simulink model "Buck_w_PI_Controller"  (R2023b)
settings: Solver=ode45  StartTime=0.0  StopTime=2.5e-5*400  MaxStep=1e-7  RelTol=1e-5
libraries: spsSeriesRLCBranchLib x3, simulink x2, spsCurrentMeasurementLib x1, spsControlledVoltageSourceLib x1, spsDiodeLib x1, spsMosfetLib x1, spsVoltageMeasurementLib x1, sps_lib x1
settings Model: Creator=jiaxinteng  LastModifiedBy=Dajr
settings SolverCC: AlgebraicLoopSolver=TrustRegion
settings DataIOCC: ReturnWorkspaceOutputs=off
settings OptimizationCC: LifeSpan=inf
settings DebuggingCC: UnconnectedInputMsg=warning  UnconnectedOutputMsg=warning  UnconnectedLineMsg=warning  SFExecutionAtInitializationDiag=none  ArithmeticOperatorsInVariantConditions=warning
settings HardwareCC: ProdBitPerSizeT=32  ProdBitPerPtrDiffT=32  ProdWordSize=32  ProdHWDeviceType=Specified
settings ModelReferenceCC: EnableRefExpFcnMdlSchedulingChecks=on
settings SFSimCC: SimUseLocalCustomCode=off  CustomCodeUndefinedFunction=UseInterfaceOnly
settings RTWCC: RTWUseLocalCustomCode=off
settings CodeAppCC: StateflowObjectComments=on
settings SimscapeCC: SimscapeNormalizeSystem=off
settings ConfigurationSet: Description=SimMechanics 2G

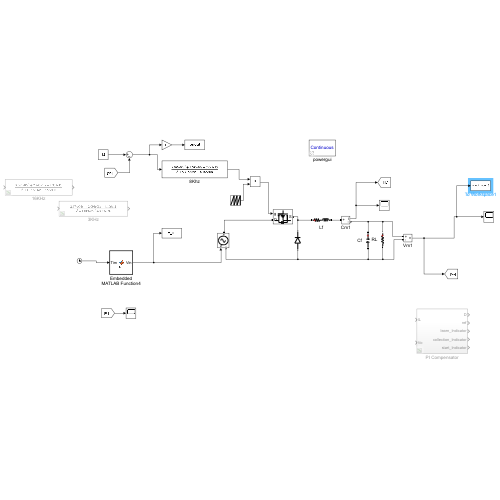
[thumbnail: Simulink's stored preview of the top-level diagram]
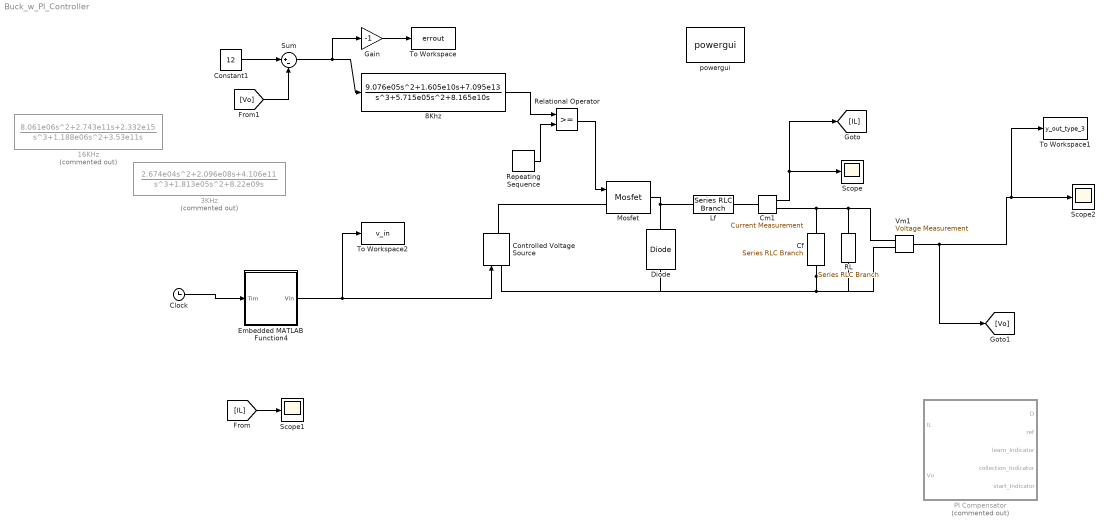
== system Buck_w_PI_Controller ==
  16KHz : TransferFcn  Commented=on  Numerator=[8.061e06 2.743e11 2.332e15]  Denominator=[1 1.188e06 3.53e11 0]
  3KHz : TransferFcn  Commented=on  Numerator=[2.674e04 2.096e08 4.106e11]  Denominator=[1 1.813e05 8.22e09 0]
  8Khz : TransferFcn  Numerator=[9.076e05 1.605e10 7.095e13]  Denominator=[1 5.715e05 8.165e10 0]
  Cf : spsSeriesRLCBranchLib/Series RLC Branch  LConnTagsString=__new0  RConnTagsString=__new0  BranchType=C  Resistance=20e-3  Inductance=220e-6  SetiL0=off  InitialCurrent=0  Capacitance=50e-6  Setx0=off  InitialVoltage=7  Measurements=None
  Clock : Clock
  Cm1 : spsCurrentMeasurementLib/Current Measurement  PhasorSimulation=off  OutputType=Complex  PSBequivalent=0
  Constant1 : Constant  Value=12
  Controlled Voltage Source : spsControlledVoltageSourceLib/Controlled Voltage Source  Initialize=on  Source_Type=AC  Amplitude=0  Phase=0  Frequency=0  Measurements=None
  Diode : spsDiodeLib/Diode  Ron=0.001  Lon=0  Vf=0.8  IC=0  UseSnubber=off  Rs=500  Cs=250e-9  Measurements=off
  Embedded MATLAB Function4 : MATLAB Function  TreatAsAtomicUnit=on  SystemSampleTime=2.5e-5
  Gain : Gain  Gain=-1
  Lf : spsSeriesRLCBranchLib/Series RLC Branch  LConnTagsString=__new0  RConnTagsString=__new0  BranchType=RL  Resistance=0.1  Inductance=220e-6  SetiL0=off  InitialCurrent=0  Capacitance=1e-6  Setx0=off  InitialVoltage=0  Measurements=None
  Mosfet : spsMosfetLib/Mosfet  Ron=0.1  Lon=0  Rd=0.01  Vfd=0  IC=0  Rs=1e5  Cs=inf  Measurements=off
  PI Compensator : Subsystem  Commented=on
  RL : spsSeriesRLCBranchLib/Series RLC Branch  LConnTagsString=__new0  RConnTagsString=__new0  BranchType=R  Resistance=10  Inductance=220e-6  SetiL0=off  InitialCurrent=0  Capacitance=50e-6  Setx0=off  InitialVoltage=0  Measurements=None
  Relational Operator : RelationalOperator  OutDataTypeStr=boolean  RndMeth=Simplest  InputSameDT=off
  Repeating Sequence : simulink/Sources/Repeating Sequence  rep_seq_t=[0 1/160000]  rep_seq_y=[0 1]
  Scope : Scope
  Scope1 : Scope
  Scope2 : Scope
  Sum : Sum  Inputs=|+-
  To Workspace : ToWorkspace  VariableName=errout  SaveFormat=Timeseries  SampleTime=-1
  To Workspace1 : ToWorkspace  VariableName=y_out_type_3  SaveFormat=Timeseries  SampleTime=-1
  To Workspace2 : ToWorkspace  VariableName=v_in  SaveFormat=Timeseries  SampleTime=-1
  Vm1 : spsVoltageMeasurementLib/Voltage Measurement  PhasorSimulation=off  OutputType=Complex  PSBequivalent=0
  powergui : sps_lib/powergui  Priority=1  SimulationMode=Continuous  SampleTime=1e-7  frequency=60  Iterations=50  frequencyindice=0  Pbase=100e6  ErrMax=1e-4  UnitsV=kV  UnitsW=MW  buscounter=0  FunctionMessages=off  echomessages=off  EnableUseOfTLC=off  CurrentSourceSwitches=off  DisableSnubberDevices=on  DisableRonSwitches=on  DisableVfSwitches=on  DisplayEquations=off  AutomaticDiscreteSolvers=off  SolverType=Tustin/Backward Euler (TBE)  Interpol=off  ExternalGateDelay=off  methode=off  Ts=10  x0status=blocks  SPID=off  SwTol=0  HookPort=off  NonlinearTolerance=1e-4  nMaxIteration=100  ContinueOnMaxIteration=off  RestoreLinks=warning  ResistiveCurrentMeasurement=off  Frange=[0:2:500]  Ylog=off  Xlog=on  ShowGrid=off  save=off  variable=ZData  structure=x1  ZoomFFT=off  StartTime=0.0  cycles=1  DisplayStyle=1  fundamental=80e3  FreqAxis=off  MaxFrequency=100e3  frequencyindicesteady=1  RmsSteady=1  display=off
  wires:
  Cm1/1 -> [IL], Scope/1
  Vm1/1 -> [Vo], To Workspace1/1, Scope2/1
  Clock/1 -> Embedded MATLAB Function4/1(Tim)
  Embedded MATLAB Function4/1(Vin) -> To Workspace2/1, Controlled Voltage Source/1
  [IL] -> Scope1/1
  Constant1/1 -> Sum/1
  [Vo] -> Sum/2
  Sum/1 -> 8Khz/1, Gain/1
  8Khz/1 -> Relational Operator/1
  Repeating Sequence/1 -> Relational Operator/2
  Relational Operator/1 -> Mosfet/1
  Gain/1 -> To Workspace/1
  connections:
  Diode/RConn1 -- Lf/LConn1 -- Mosfet/RConn1
  Vm1/LConn1 -- RL/LConn1 -- Cm1/RConn1 -- Cf/LConn1
  Cf/RConn1 -- Vm1/LConn2 -- RL/RConn1 -- Controlled Voltage Source/LConn1 -- Diode/LConn1
  Cm1/LConn1 -- Lf/RConn1
  Mosfet/LConn1 -- Controlled Voltage Source/RConn1

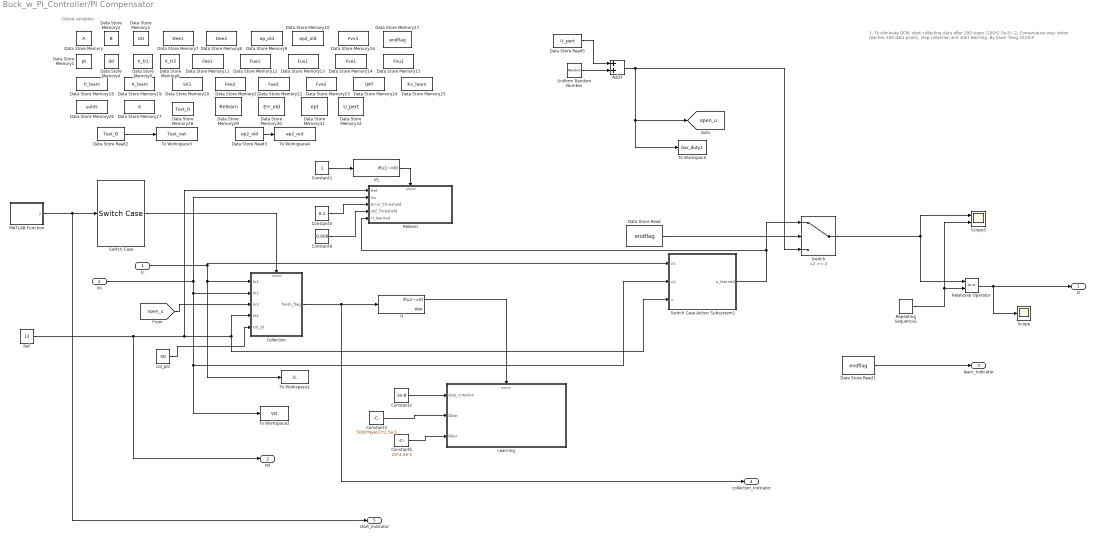
== system Buck_w_PI_Controller/PI Compensator ==
  note: Global variables:
  note: 1. To eliminate DCM, start collecting data after 200 steps (200*2.5e-5),
      | 2. Conservative way: when reaches 100 data points, stop collection and start learning.
      |
      | By Jiaxin Teng
      | 2019.8
  IL : Inport
  Vo : Inport  Port=2
  Add3 : Sum
  Collection : Subsystem  TreatAsAtomicUnit=on
  Constant1 : Constant
  Constant2 : Constant  Value=1e-8
  Constant3 : Constant  Value=5000*eye(2)*2.5e-5
  Constant4 : Constant  Value=20*2.5e-5
  Constant5 : Constant  Value=0.1
  Constant6 : Constant  Value=0.008
  Data Store Memory : DataStoreMemory  ReadBeforeWriteMsg=warning  WriteAfterWriteMsg=warning  WriteAfterReadMsg=warning  InitialValue=zeros(50,1)  ShowAdditionalParam=off  OutDataTypeStr=double
  Data Store Memory1 : DataStoreMemory  DataStoreName=pt  ReadBeforeWriteMsg=warning  WriteAfterWriteMsg=warning  WriteAfterReadMsg=warning  InitialValue=1  ShowAdditionalParam=off  OutDataTypeStr=double
  Data Store Memory10 : DataStoreMemory  DataStoreName=ep2_old  ReadBeforeWriteMsg=warning  WriteAfterWriteMsg=warning  WriteAfterReadMsg=warning  InitialValue=zeros(1,2)  VectorParams1D=off  ShowAdditionalParam=off  OutDataTypeStr=double
  Data Store Memory11 : DataStoreMemory  DataStoreName=Fee1  ReadBeforeWriteMsg=warning  WriteAfterWriteMsg=warning  WriteAfterReadMsg=warning  InitialValue=zeros(50,4)  ShowAdditionalParam=off  OutDataTypeStr=double
  Data Store Memory12 : DataStoreMemory  DataStoreName=Fue1  ReadBeforeWriteMsg=warning  WriteAfterWriteMsg=warning  WriteAfterReadMsg=warning  InitialValue=zeros(50,2)  ShowAdditionalParam=off  OutDataTypeStr=double
  Data Store Memory13 : DataStoreMemory  DataStoreName=Fuu1  ReadBeforeWriteMsg=warning  WriteAfterWriteMsg=warning  WriteAfterReadMsg=warning  InitialValue=zeros(50,1)  ShowAdditionalParam=off  OutDataTypeStr=double
  Data Store Memory14 : DataStoreMemory  DataStoreName=Fve1  ReadBeforeWriteMsg=warning  WriteAfterWriteMsg=warning  WriteAfterReadMsg=warning  InitialValue=zeros(50,2)  ShowAdditionalParam=off  OutDataTypeStr=double
  Data Store Memory15 : DataStoreMemory  DataStoreName=Fvu1  ReadBeforeWriteMsg=warning  WriteAfterWriteMsg=warning  WriteAfterReadMsg=warning  InitialValue=zeros(50,1)  ShowAdditionalParam=off  OutDataTypeStr=double
  Data Store Memory16 : DataStoreMemory  DataStoreName=Fvv1  ReadBeforeWriteMsg=warning  WriteAfterWriteMsg=warning  WriteAfterReadMsg=warning  InitialValue=zeros(50,1)  ShowAdditionalParam=off  OutDataTypeStr=double
  Data Store Memory17 : DataStoreMemory  DataStoreName=endflag  ReadBeforeWriteMsg=warning  WriteAfterWriteMsg=warning  WriteAfterReadMsg=warning  ShowAdditionalParam=off  OutDataTypeStr=double
  Data Store Memory18 : DataStoreMemory  DataStoreName=P_learn  ReadBeforeWriteMsg=warning  WriteAfterWriteMsg=warning  WriteAfterReadMsg=warning  InitialValue=zeros(2,2)  ShowAdditionalParam=off  OutDataTypeStr=double
  Data Store Memory19 : DataStoreMemory  DataStoreName=K_learn  ReadBeforeWriteMsg=warning  WriteAfterWriteMsg=warning  WriteAfterReadMsg=warning  InitialValue=zeros(1,2)  VectorParams1D=off  ShowAdditionalParam=off  OutDataTypeStr=double
  Data Store Memory2 : DataStoreMemory  DataStoreName=B  ReadBeforeWriteMsg=warning  WriteAfterWriteMsg=warning  WriteAfterReadMsg=warning  InitialValue=zeros(50,1)  ShowAdditionalParam=off  OutDataTypeStr=double
  Data Store Memory20 : DataStoreMemory  DataStoreName=SX1  ReadBeforeWriteMsg=warning  WriteAfterWriteMsg=warning  WriteAfterReadMsg=warning  InitialValue=zeros(2,1)  ShowAdditionalParam=off  OutDataTypeStr=double
  Data Store Memory21 : DataStoreMemory  DataStoreName=Fee2  ReadBeforeWriteMsg=warning  WriteAfterWriteMsg=warning  WriteAfterReadMsg=warning  InitialValue=zeros(50,4)  ShowAdditionalParam=off  OutDataTypeStr=double
  Data Store Memory22 : DataStoreMemory  DataStoreName=Fue2  ReadBeforeWriteMsg=warning  WriteAfterWriteMsg=warning  WriteAfterReadMsg=warning  InitialValue=zeros(50,2)  ShowAdditionalParam=off  OutDataTypeStr=double
  Data Store Memory23 : DataStoreMemory  DataStoreName=Fve2  ReadBeforeWriteMsg=warning  WriteAfterWriteMsg=warning  WriteAfterReadMsg=warning  InitialValue=zeros(50,2)  ShowAdditionalParam=off  OutDataTypeStr=double
  Data Store Memory24 : DataStoreMemory  DataStoreName=QKf  ReadBeforeWriteMsg=warning  WriteAfterWriteMsg=warning  WriteAfterReadMsg=warning  InitialValue=zeros(2,2)  ShowAdditionalParam=off  OutDataTypeStr=double
  Data Store Memory25 : DataStoreMemory  DataStoreName=Kv_learn  ReadBeforeWriteMsg=warning  WriteAfterWriteMsg=warning  WriteAfterReadMsg=warning  ShowAdditionalParam=off  OutDataTypeStr=double
  Data Store Memory26 : DataStoreMemory  DataStoreName=sol45  ReadBeforeWriteMsg=warning  WriteAfterWriteMsg=warning  WriteAfterReadMsg=warning  InitialValue=zeros(2,1)  ShowAdditionalParam=off  OutDataTypeStr=double
  Data Store Memory27 : DataStoreMemory  DataStoreName=K  ReadBeforeWriteMsg=warning  WriteAfterWriteMsg=warning  WriteAfterReadMsg=warning  InitialValue=[0.2,0.2]  VectorParams1D=off  ShowAdditionalParam=off  OutDataTypeStr=double
  Data Store Memory28 : DataStoreMemory  DataStoreName=Test_D  ReadBeforeWriteMsg=warning  WriteAfterWriteMsg=warning  WriteAfterReadMsg=warning  InitialValue=zeros(50,4)  ShowAdditionalParam=off  OutDataTypeStr=double
  Data Store Memory29 : DataStoreMemory  DataStoreName=Relearn  ReadBeforeWriteMsg=warning  WriteAfterWriteMsg=warning  WriteAfterReadMsg=warning  ShowAdditionalParam=off  OutDataTypeStr=double
  Data Store Memory3 : DataStoreMemory  DataStoreName=UU  ReadBeforeWriteMsg=warning  WriteAfterWriteMsg=warning  WriteAfterReadMsg=warning  InitialValue=zeros(50,1)  ShowAdditionalParam=off  OutDataTypeStr=double
  Data Store Memory30 : DataStoreMemory  DataStoreName=Err_old  ReadBeforeWriteMsg=warning  WriteAfterWriteMsg=warning  WriteAfterReadMsg=warning  InitialValue=zeros(1000,1)  ShowAdditionalParam=off  OutDataTypeStr=double
  Data Store Memory31 : DataStoreMemory  DataStoreName=ept  ReadBeforeWriteMsg=warning  WriteAfterWriteMsg=warning  WriteAfterReadMsg=warning  InitialValue=1  ShowAdditionalParam=off  OutDataTypeStr=double
  Data Store Memory32 : DataStoreMemory  DataStoreName=U_pert  ReadBeforeWriteMsg=warning  WriteAfterWriteMsg=warning  WriteAfterReadMsg=warning  InitialValue=0.32  ShowAdditionalParam=off  OutDataTypeStr=double
  Data Store Memory4 : DataStoreMemory  DataStoreName=dd  ReadBeforeWriteMsg=warning  WriteAfterWriteMsg=warning  WriteAfterReadMsg=warning  InitialValue=1  ShowAdditionalParam=off  OutDataTypeStr=uint8
  Data Store Memory5 : DataStoreMemory  DataStoreName=X_tr1  ReadBeforeWriteMsg=warning  WriteAfterWriteMsg=warning  WriteAfterReadMsg=warning  InitialValue=[0;1]  ShowAdditionalParam=off  OutDataTypeStr=double
  Data Store Memory6 : DataStoreMemory  DataStoreName=X_tr2  ReadBeforeWriteMsg=warning  WriteAfterWriteMsg=warning  WriteAfterReadMsg=warning  InitialValue=[1;0]  ShowAdditionalParam=off  OutDataTypeStr=double
  Data Store Memory7 : DataStoreMemory  DataStoreName=Dee1  ReadBeforeWriteMsg=warning  WriteAfterWriteMsg=warning  WriteAfterReadMsg=warning  InitialValue=zeros(50,3)  ShowAdditionalParam=off  OutDataTypeStr=double
  Data Store Memory8 : DataStoreMemory  DataStoreName=Dee2  ReadBeforeWriteMsg=warning  WriteAfterWriteMsg=warning  WriteAfterReadMsg=warning  InitialValue=zeros(50,3)  ShowAdditionalParam=off  OutDataTypeStr=double
  Data Store Memory9 : DataStoreMemory  DataStoreName=ep_old  ReadBeforeWriteMsg=warning  WriteAfterWriteMsg=warning  WriteAfterReadMsg=warning  InitialValue=zeros(1,2)  VectorParams1D=off  ShowAdditionalParam=off  OutDataTypeStr=double
  Data Store Read : DataStoreRead  DataStoreName=endflag  IndexOptions=Index vector (dialog)  Indices=1  OutputSizes=1
  Data Store Read1 : DataStoreRead  DataStoreName=endflag  IndexOptions=Index vector (dialog)  Indices=1  OutputSizes=1
  Data Store Read2 : DataStoreRead  DataStoreName=Test_D  IndexOptions=Index vector (dialog)  Indices=1  OutputSizes=1
  Data Store Read3 : DataStoreRead  DataStoreName=ep2_old  IndexOptions=Index vector (dialog)  Indices=1  OutputSizes=1
  Data Store Read5 : DataStoreRead  DataStoreName=U_pert  IndexOptions=Index vector (dialog)  Indices=1  OutputSizes=1
  If : If  IfExpression=u1~=0
  If1 : If  IfExpression=u1~=0  ShowElse=off
  Learning : Subsystem  TreatAsAtomicUnit=on
  MATLAB Function : MATLAB Function  TreatAsAtomicUnit=on  SystemSampleTime=2.5e-5
  Ref : Constant  Value=12
  Relational Operator : RelationalOperator  OutDataTypeStr=boolean  InputSameDT=off
  Relearn : Subsystem
  Repeating Sequence1 : simulink/Sources/Repeating Sequence  rep_seq_t=[0 1/(160e3) 1/(80e3)]  rep_seq_y=[0 1 0]
  Scope : Scope
  Scope3 : Scope  NumInputPorts=2
  Switch : Switch  Threshold=2  SaturateOnIntegerOverflow=off  InputSameDT=off
  Switch Case : SwitchCase  CaseConditions={1,2}
  Switch Case Action Subsystem1 : Subsystem  TreatAsAtomicUnit=on
  To Workspace : ToWorkspace  VariableName=bar_duty1  SaveFormat=Structure With Time  SampleTime=2.5e-5
  To Workspace1 : ToWorkspace  VariableName=IL  SaveFormat=Structure With Time  SampleTime=2.5e-5
  To Workspace2 : ToWorkspace  VariableName=VO  SaveFormat=Structure With Time  SampleTime=2.5e-5
  To Workspace3 : ToWorkspace  VariableName=Test_out  SaveFormat=Timeseries  SampleTime=-1
  To Workspace4 : ToWorkspace  VariableName=ep2_out  SaveFormat=Timeseries  SampleTime=-1
  Uniform Random Number : UniformRandomNumber  Minimum=-5e-3  Maximum=5e-3  SampleTime=2.5e-5
  col_pts : Constant  Value=50
  D : Outport
  ref : Outport  Port=2
  learn_Indicator : Outport  Port=3
  collection_Indicator : Outport  Port=4
  start_Indicator : Outport  Port=5
  tag scope: open_u=global
  wires:
  Relational Operator/1 -> D/1, Scope/1
  Repeating Sequence1/1 -> Scope3/2, Relational Operator/2
  IL/1 -> To Workspace1/1, Collection/1(In1), Switch Case Action Subsystem1/1(x1)
  Vo/1 -> To Workspace2/1, Switch Case Action Subsystem1/2(x2), Collection/2(In2), Relearn/2(Vo)
  Collection/1(finish_flag) -> collection_Indicator/1, If/1
  If/1 -> Learning/Action
  [open_u] -> Collection/3(In3)
  Switch Case/2 -> Collection/Action
  MATLAB Function/1(y) -> start_Indicator/1, Switch Case/1
  Constant2/1 -> Learning/1(stop_criterion)
  Constant3/1 -> Learning/2(Qbar)
  Constant4/1 -> Learning/3(Rbar)
  Data Store Read/1 -> Switch/2
  Switch Case Action Subsystem1/1(u_learned) -> Relearn/5(U_learned), Switch/1
  Add3/1 -> [open_u], To Workspace/1, Switch/3
  Switch/1 -> Scope3/1, Relational Operator/1
  Data Store Read5/1 -> Add3/1
  Uniform Random Number/1 -> Add3/2
  Data Store Read1/1 -> learn_Indicator/1
  Data Store Read3/1 -> To Workspace4/1
  Data Store Read2/1 -> To Workspace3/1
  Constant5/1 -> Relearn/3(Error_Threshold)
  Constant6/1 -> Relearn/4(std_Threshold)
  Ref/1 -> ref/1, Relearn/1(Ref), Collection/4(In4), Switch Case Action Subsystem1/3(v)
  If1/1 -> Relearn/Action
  Constant1/1 -> If1/1
  col_pts/1 -> Collection/5(col_pt)

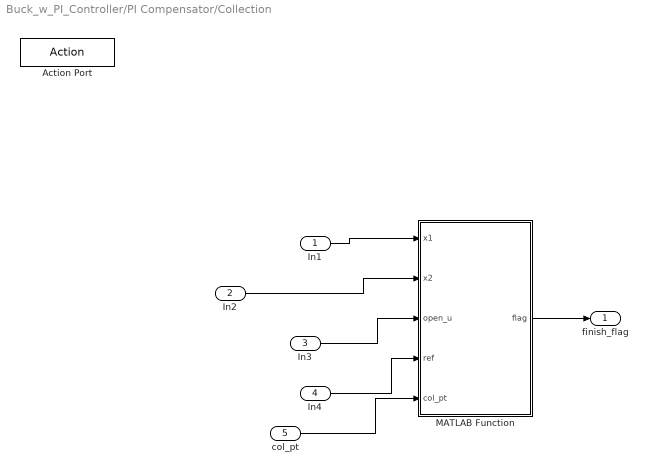
== system Buck_w_PI_Controller/PI Compensator/Collection ==
  In1 : Inport
  In2 : Inport  Port=2
  In3 : Inport  Port=3
  In4 : Inport  Port=4
  col_pt : Inport  Port=5
  Action Port : ActionPort  ActionPortLabel=case [ 2 ]:
  MATLAB Function : MATLAB Function  TreatAsAtomicUnit=on  SystemSampleTime=2.5e-5
  finish_flag : Outport
  wires:
  In1/1 -> MATLAB Function/1(x1)
  In2/1 -> MATLAB Function/2(x2)
  In3/1 -> MATLAB Function/3(open_u)
  MATLAB Function/1(flag) -> finish_flag/1
  In4/1 -> MATLAB Function/4(ref)
  col_pt/1 -> MATLAB Function/5(col_pt)

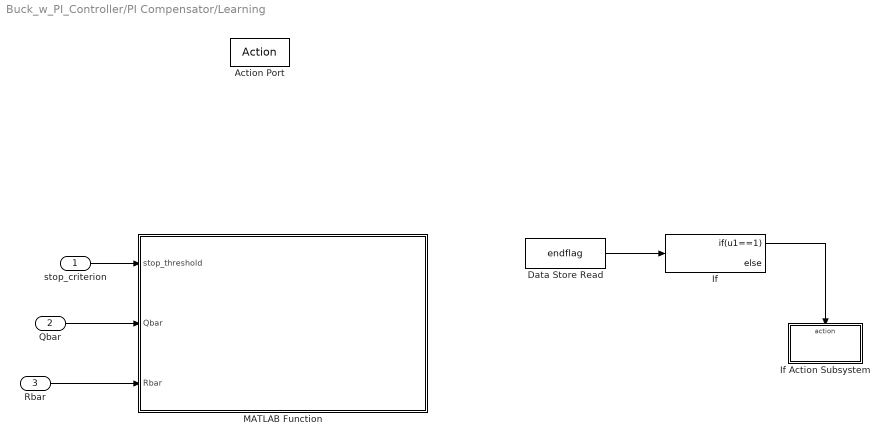
== system Buck_w_PI_Controller/PI Compensator/Learning ==
  stop_criterion : Inport
  Qbar : Inport  Port=2
  Rbar : Inport  Port=3
  Action Port : ActionPort  ActionPortLabel=if(u1~=0)
  Data Store Read : DataStoreRead  DataStoreName=endflag  IndexOptions=Index vector (dialog)  Indices=1  OutputSizes=1
  If : If  IfExpression=u1==1
  If Action Subsystem : Subsystem  TreatAsAtomicUnit=on
  MATLAB Function : MATLAB Function  TreatAsAtomicUnit=on
  wires:
  stop_criterion/1 -> MATLAB Function/1(stop_threshold)
  Data Store Read/1 -> If/1
  If/1 -> If Action Subsystem/Action
  Qbar/1 -> MATLAB Function/2(Qbar)
  Rbar/1 -> MATLAB Function/3(Rbar)

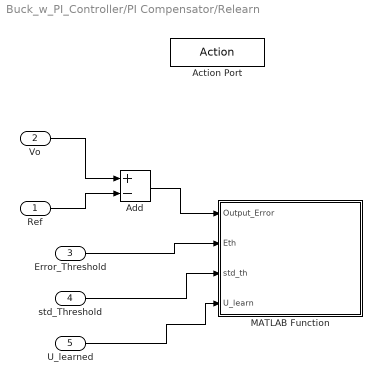
== system Buck_w_PI_Controller/PI Compensator/Relearn ==
  Ref : Inport
  Vo : Inport  Port=2
  Error_Threshold : Inport  Port=3
  std_Threshold : Inport  Port=4
  U_learned : Inport  Port=5
  Action Port : ActionPort  ActionPortLabel=if(u1~=0)
  Add : Sum  Inputs=+-
  MATLAB Function : MATLAB Function  TreatAsAtomicUnit=on
  wires:
  Error_Threshold/1 -> MATLAB Function/2(Eth)
  std_Threshold/1 -> MATLAB Function/3(std_th)
  Ref/1 -> Add/2
  Vo/1 -> Add/1
  Add/1 -> MATLAB Function/1(Output_Error)
  U_learned/1 -> MATLAB Function/4(U_learn)

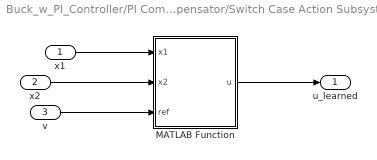
== system Buck_w_PI_Controller/PI Compensator/Switch Case Action Subsystem1 ==
  x1 : Inport
  x2 : Inport  Port=2
  v : Inport  Port=3
  MATLAB Function : MATLAB Function  TreatAsAtomicUnit=on  SystemSampleTime=2.5e-5
  u_learned : Outport
  wires:
  x1/1 -> MATLAB Function/1(x1)
  x2/1 -> MATLAB Function/2(x2)
  v/1 -> MATLAB Function/3(ref)
  MATLAB Function/1(u) -> u_learned/1

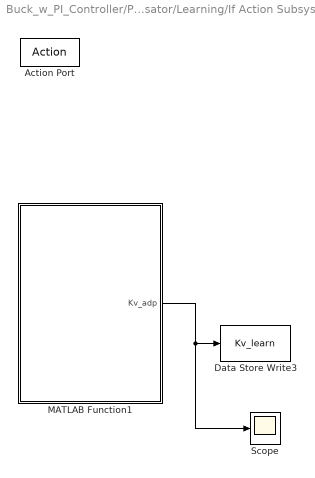
== system Buck_w_PI_Controller/PI Compensator/Learning/If Action Subsystem ==
  Action Port : ActionPort  ActionPortLabel=if(u1==1)
  Data Store Write3 : DataStoreWrite  DataStoreName=Kv_learn  IndexOptions=Index vector (dialog)  Indices=1  OutputSizes=1
  MATLAB Function1 : MATLAB Function  TreatAsAtomicUnit=on
  Scope : Scope
  wires:
  MATLAB Function1/1(Kv_adp) -> Scope/1, Data Store Write3/1

== matlab function Buck_w_PI_Controller/PI Compensator/Learning/If Action Subsystem/MATLAB Function1 ==
  data: Dee1 data_store_memory; Dee2 data_store_memory; Fee2 data_store_memory; Fue2 data_store_memory; Fve2 data_store_memory; Fvu1 data_store_memory; Fuu1 data_store_memory; Fvv1 data_store_memory; Kv_adp output; endflag data_store_memory; QKf data_store_memory; X_tr1 data_store_memory; X_tr2 data_store_memory; K_learn data_store_memory; SX1 data_store_memory; sol45 data_store_memory
function Kv_adp  = fcn
global Dee2 Fee2 Fue2 Fve2 Fvu1 Fuu1 Fvv1 K_learn SX1 endflag QKf X_tr1 X_tr2 sol45


    phi12=Dee2(2:end,:);
    Y2=Fee2(1:end-1,:)*QKf(:); 
    phi22=-2*((Fee2(1:end-1,:)*kron(K_learn',eye(2)))+Fue2(1:end-1,:));
    phi32=-Fuu1(1:end-1,:)+Fee2(1:end-1,:)*kron(K_learn',K_learn');
    phi42=-Fvv1(1:end-1,:);
    phi52=2*Fve2(1:end-1,:);
    phi62=2*Fvu1(1:end-1);
    X2=[phi12 phi22 phi32 phi42 phi52 phi62];
    sol2=(X2'*X2)\X2'*Y2;
    SX2=sol2(8:9);
    
    AA=[SX2(:) zeros(2,2) -sol45;
    X_tr2 -eye(2,2) zeros(2,1)];
    BB=[-SX1(:); -X_tr1];
    RegSol=AA\BB;
    Xreal=RegSol(2:3);
    Ureal=RegSol(4);
    Kv_adp=Ureal+K_learn*Xreal;
    endflag=2;


end

== matlab function Buck_w_PI_Controller/PI Compensator/Switch Case Action Subsystem1/MATLAB Function ==
  data: x1 input; u output; x2 input; ref input; K_learn data_store_memory; Kv_learn data_store_memory
function u = fcn(x1,x2,ref)
global K_learn Kv_learn

u=-K_learn*[x1;x2]+Kv_learn*ref;

if(u>1)
    u=1;
elseif(u<0)
    u=0;
end

end

== matlab function Buck_w_PI_Controller/PI Compensator/Relearn/MATLAB Function ==
  data: Output_Error input; Eth input; std_th input; endflag data_store_memory; pt data_store_memory; ept data_store_memory; Relearn data_store_memory; Err_old data_store_memory; U_learn input; U_pert data_store_memory
function fcn(Output_Error, Eth, std_th, U_learn)
global endflag pt Relearn Err_old ept U_pert

Err_old(ept) = Output_Error;
ept = ept+1;
if ept>(length(Err_old))
    ept=ept-(length(Err_old));
end
err_mean = mean(Err_old);
err_std = std(Err_old);

if ( (abs(err_mean) > Eth) && (err_std < std_th) ) && ( (endflag == 2)&& (Relearn == 0) )
    U_pert = U_learn;
    pt=1;
    endflag=0;

end

end

== matlab function Buck_w_PI_Controller/Embedded MATLAB Function4 ==
  data: Vin output; Tim input
function Vin = fcn(Tim)  

Vin=40;

% if (Tim>0.009)&&(Tim<0.01275)
%     Vin=48;
% elseif (Tim>=0.01275)&&(Tim<0.0163)
%     Vin=60;
% elseif (Tim>=0.0163)
%     Vin=36;
% end

end

== matlab function Buck_w_PI_Controller/PI Compensator/Learning/MATLAB Function ==
  data: Dee1 data_store_memory; Dee2 data_store_memory; Fee1 data_store_memory; Fue1 data_store_memory; Fve1 data_store_memory; Fvu1 data_store_memory; Fuu1 data_store_memory; Fvv1 data_store_memory; endflag data_store_memory; stop_threshold input; QKf data_store_memory; sol45 data_store_memory; P_learn data_store_memory; K_learn data_store_memory; SX1 data_store_memory; Qbar input; Rbar input; K data_store_memory
function fcn(stop_threshold,Qbar,Rbar)
global Dee1 Fee1 Fue1 Fve1 Fvu1 Fuu1 Fvv1 endflag QKf sol45 P_learn K_learn SX1 K
    
phi1=Dee1(2:end,:); Pp=zeros(2); 


%for m=1:50
while endflag==0
QK=-Qbar-K'*Rbar*K;

phi2=-2*((Fee1(1:end-1,:)*kron(K',eye(2)))+Fue1(1:end-1,:));
phi3=-Fuu1(1:end-1)+Fee1(1:end-1,:)*kron(K',K');
phi4=-Fvv1(1:end-1);
phi5=2*Fve1(1:end-1,:);
phi6=2*Fvu1(1:end-1);

X=[phi1 phi2 phi3 phi4 phi5 phi6];

% RANK=rank(X);
    
Y=Fee1(1:end-1,:)*QK(:);

sol=(X'*X)\X'*Y;

P=[sol(1) sol(2)/2; sol(2)/2 sol(3)];
K=(Rbar+sol(6))\sol(4:5)';

if(norm(P-Pp)<stop_threshold)
    P_learn=P; K_learn=K; SX1=sol(8:9); QKf=-Qbar-K'*Rbar*K; sol45=sol(4:5);
    endflag=1;
else 
    endflag=0;
end

Pp=P;

end

end

== matlab function Buck_w_PI_Controller/PI Compensator/Collection/MATLAB Function ==
  data: x1 input; pt data_store_memory; A data_store_memory; flag output; x2 input; B data_store_memory; open_u input; UU data_store_memory; X_tr1 data_store_memory; X_tr2 data_store_memory; Dee1 data_store_memory; Dee2 data_store_memory; ref input; ep_old data_store_memory; ep2_old data_store_memory; Fee1 data_store_memory; Fue1 data_store_memory; Fve1 data_store_memory; Fvu1 data_store_memory; Fuu1 data_store_memory; Fvv1 data_store_memory; Fee2 data_store_memory; Fve2 data_store_memory; Fue2 data_store_memory; Test_D data_store_memory; Relearn data_store_memory; col_pt input
function flag=fcn(x1,x2,open_u,ref, col_pt)
global A B UU pt X_tr1 X_tr2 Dee1 Dee2 Fee1 Fee2 Fue1 Fue2 Fve1...
    Fve2 Fvu1 Fuu1 Fvv1 ep_old ep2_old Test_D Relearn

flag=0;

X_open=[x1 x2];

ep=X_open-ref*X_tr1';
ep2=X_open-ref*X_tr2';
dee1=kron(ep,ep)-kron(ep_old,ep_old);
dee2=kron(ep2,ep2)-kron(ep2_old,ep2_old);
fee1=kron(ep,ep);
fee2=kron(ep2,ep2);
fue1=kron(open_u,ep);
fue2=kron(open_u,ep2);
fve1=kron(ref,ep);
fve2=kron(ref,ep2);
fvu1=kron(ref,open_u);
fuu1=kron(open_u,open_u);

if pt<(col_pt+1)         % if the indicator doesn't show 100 points has been reached, keep on collecting
    %A(pt)=x1;
    %B(pt)=x2;
    %UU(pt)=open_u;
    Relearn =1;
    Test_D(pt,:)=dee1(:,:);
    Dee1(pt,:)=dee1(:,[1,2,4]);
    Dee2(pt,:)=dee2(:,[1,2,4]);
    Fee1(pt,:)=fee1;
    Fee2(pt,:)=fee2;
    Fue1(pt,:)=fue1;
    Fue2(pt,:)=fue2;
    Fve1(pt,:)=fve1;
    Fve2(pt,:)=fve2;
    Fvu1(pt,:)=fvu1;
    Fuu1(pt,:)=fuu1;
    Fvv1(pt,:)=ref;
    
    pt=pt+1;
end
ep_old=ep;
ep2_old=ep2;

       
        
        %Fee1=kron(ep,ep);
        %Fue1=kron(un,ep);
        %Fuu1=kron(un,un);
        %Fvv1=kron(Ar,Ar);
        %Fve1=kron(Ar,ep);
        %Fvu1=kron(Ar,un); 

    

if pt>=(col_pt+1)
    flag=1;
    Relearn=0;
    pt=(col_pt+1);
end



end

== matlab function Buck_w_PI_Controller/PI Compensator/MATLAB Function ==
  data: y output; dd data_store_memory
function y = fcn
global dd

if dd<=200
    y=1;
    dd=dd+1;
else
    y=2;
end

end
